simulink subsystem "CSROpDecoder"  (R2024b)
settings: Solver=VariableStepAuto  StartTime=0.0  StopTime=10.0  RelTol=1e-3
settings Model: Creator=stefano  LastModifiedBy=stefano

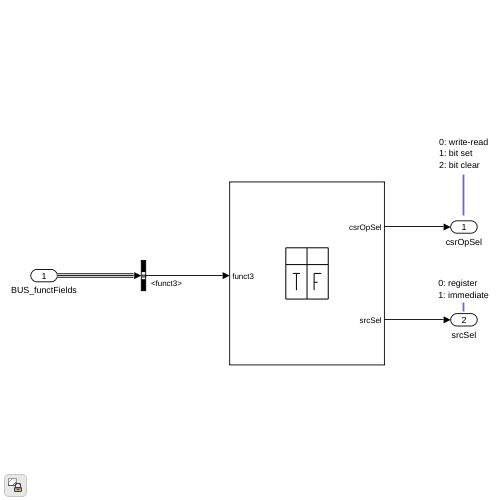
[thumbnail: Simulink's stored preview of the top-level diagram]
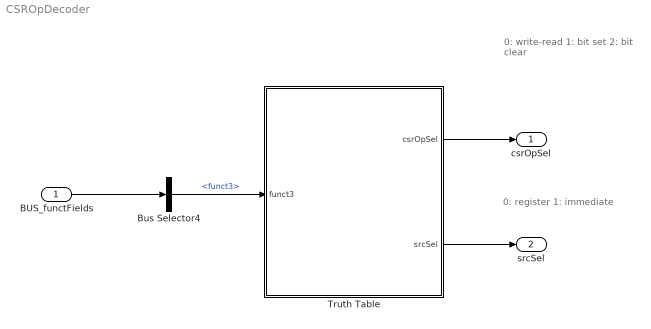
== system CSROpDecoder ==
  note: 0: write-read
      | 1: bit set
      | 2: bit clear
  note: 0: register
      | 1: immediate
  BUS_functFields : Inport
  Bus Selector4 : BusSelector  OutputSignals=funct3
  Truth Table : Truth Table  TreatAsAtomicUnit=on
  csrOpSel : Outport
  srcSel : Outport  Port=2
  wires:
  BUS_functFields/1 -> Bus Selector4/1
  Bus Selector4/1 -> Truth Table/1(funct3)  "<funct3>"
  Truth Table/1(csrOpSel) -> csrOpSel/1
  Truth Table/2(srcSel) -> srcSel/1

== matlab function CSROpDecoder/Truth Table ==
  data: funct3 input; csrOpSel output fixdt(0,2,0); srcSel output boolean
function [csrOpSel, srcSel] = fcn(funct3)

aVarTruthTableCondition_1 = false;
aVarTruthTableCondition_2 = false;
aVarTruthTableCondition_3 = false;
aVarTruthTableCondition_4 = false;
aVarTruthTableCondition_5 = false;
aVarTruthTableCondition_6 = false;
aVarTruthTableCondition_7 = false;


% csrrw

aVarTruthTableCondition_1 = logical(funct3 == 1);

% csrrs

aVarTruthTableCondition_2 = logical(funct3 == 2);

% csrrc

aVarTruthTableCondition_3 = logical(funct3 == 3);

% csrrwi

aVarTruthTableCondition_4 = logical(funct3 == 5);

% csrrsi

aVarTruthTableCondition_5 = logical(funct3 == 6);

% csrrci

aVarTruthTableCondition_6 = logical(funct3 == 7);

% ecall

aVarTruthTableCondition_7 = logical(funct3 == 0);

if (aVarTruthTableCondition_1)
    csrrw();
elseif (aVarTruthTableCondition_2)
    csrrs();
elseif (aVarTruthTableCondition_3)
    csrrc();
elseif (aVarTruthTableCondition_4)
    csrrwi();
elseif (aVarTruthTableCondition_5)
    csrrsi();
elseif (aVarTruthTableCondition_6)
    csrrci();
elseif (aVarTruthTableCondition_7)
    ecall();
else % Default
    DA();
end

function DA()

% default action (should never reach)

csrOpSel = 0;
srcSel = false;

function csrrw()

% csrrw

csrOpSel = 0;
srcSel = false;

function csrrs()

% csrrs

csrOpSel = 1;
srcSel = false;

function csrrc()

% csrrc

csrOpSel = 2;
srcSel = false;

function csrrwi()

% csrrwi

csrOpSel = 0;
srcSel = true;

function csrrsi()

% csrrsi

csrOpSel = 1;
srcSel = true;

function csrrci()

% csrrci

csrOpSel = 2;
srcSel = true;

function ecall()

% ecall

csrOpSel = 2;
srcSel = true;
